simulink model "decentralized"  (R2017a)
settings: Solver=VariableStepAuto  StartTime=0.0  StopTime=6.01  RelTol=1e-3
values from neighbouring files (symbols this model uses):
  Kd = diag (Kd)    [calcula_ganhos.m]    (also in trajectoria_final.mat = [10.6713619257 0 0 0 0 0 0 10.022937202 0 0 0 0 ... (36 elem; trajectoria_final_2speed.mat = [10.6713619257 0 0 0 0 0 0 10.022937202 0 0 0 0 ... (36 elem; trajectoria_final_maxspeed.mat = [10.6713619257 0 0 0 0 0 0 10.022937202 0 0 0 0 ... (36 elem)
  Kp = diag (Kp)    [calcula_ganhos.m]    (also in trajectoria_final.mat = [67.0501444592 0 0 0 0 0 0 62.9759717625 0 0 0 0 ... (36 ele; trajectoria_final_2speed.mat = [67.0501444592 0 0 0 0 0 0 62.9759717625 0 0 0 0 ... (36 ele; trajectoria_final_maxspeed.mat = [67.0501444592 0 0 0 0 0 0 62.9759717625 0 0 0 0 ... (36 ele)
  q0 = [1.382 1.2 0.2 -0.5 0.4 0.34]'    [linear_trajectoryP.m]    (also in trajectoria_final.mat = [1.382 1.2 0.2 -0.5 0.4 0.34]; trajectoria_final_2speed.mat = [1.382 1.2 0.2 -0.5 0.4 0.34]; trajectoria_final_maxspeed.mat = [1.382 1.2 0.2 -0.5 0.4 0.34])
libraries: simulink x18, UR3_Lib x3, dspindex x2, sharedtransform x1, dspinverses x1
settings Model: Creator=dscat  LastModifiedBy=dscat

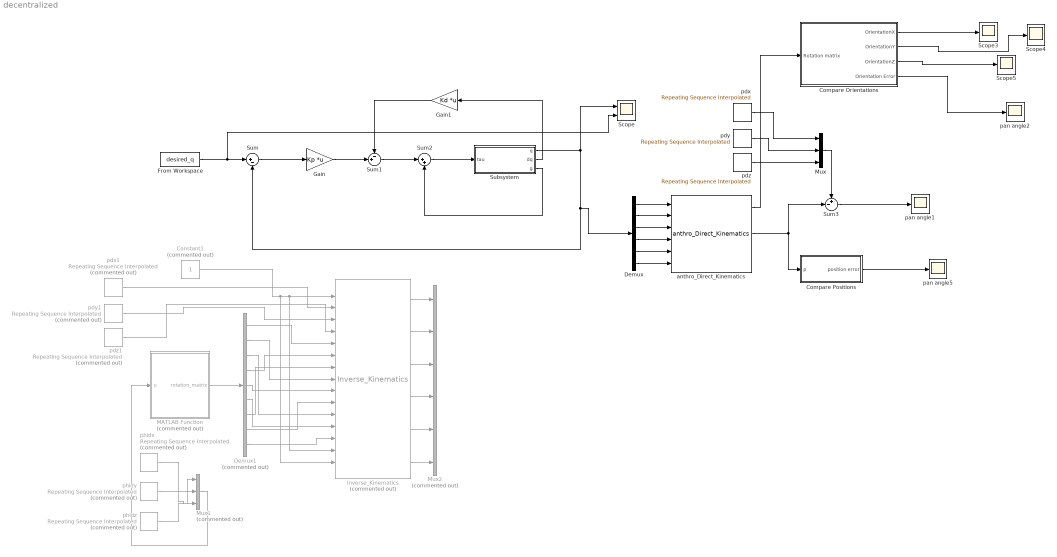
== system decentralized ==
  Compare Orientations : Subsystem
  Compare Positions : Subsystem
  Constant1 : Constant  Commented=on
  Demux : Demux  Outputs=6
  Demux1 : Demux  Commented=on  Outputs=9
  From Workspace : FromWorkspace  VariableName=desired_q  OutDataTypeStr=double  SampleTime=0
  Gain : Gain  Gain=Kp  Multiplication=Matrix(K*u)
  Gain1 : Gain  Gain=Kd  Multiplication=Matrix(K*u)
  Inverse_Kinematics : UR3_Lib/Inverse_Kinematics  Commented=on
  MATLAB Function : MATLAB Function  Commented=on  TreatAsAtomicUnit=on
  Mux : Mux  Inputs=3
  Mux1 : Mux  Commented=on  Inputs=3
  Mux2 : Mux  Commented=on  Inputs=6
  Scope : Scope  NumInputPorts=2
  Scope3 : Scope
  Scope4 : Scope
  Scope5 : Scope
  Subsystem : Subsystem
  Sum : Sum  Inputs=|+-
  Sum1 : Sum  Inputs=-+|
  Sum2 : Sum  Inputs=|++
  Sum3 : Sum  Inputs=+-|
  anthro_Direct_Kinematics : UR3_Lib/anthro_Direct_Kinematics
  pan angle1 : Scope
  pan angle2 : Scope
  pan angle5 : Scope
  pdx : simulink/Sources/Repeating Sequence Interpolated  OutValues=pdx  TimeValues=t  LookUpMeth=Interpolation-Use End Values  tsamp=0.01  OutMin=[]  OutMax=[]  OutDataTypeStr=double  OutputDataTypeScalingMode=double  OutDataType=fixdt(0,8)  OutScaling=2^-10
  pdx1 : simulink/Sources/Repeating Sequence Interpolated  Commented=on  OutValues=pdx  TimeValues=t  LookUpMeth=Interpolation-Use End Values  tsamp=0.01  OutMin=[]  OutMax=[]  OutDataTypeStr=double  OutputDataTypeScalingMode=double  OutDataType=fixdt(0,8)  OutScaling=2^-10
  pdy : simulink/Sources/Repeating Sequence Interpolated  OutValues=pdy  TimeValues=t  LookUpMeth=Interpolation-Use End Values  tsamp=0.01  OutMin=[]  OutMax=[]  OutDataTypeStr=double  OutputDataTypeScalingMode=double  OutDataType=fixdt(0,8)  OutScaling=2^-10
  pdy1 : simulink/Sources/Repeating Sequence Interpolated  Commented=on  OutValues=pdy  TimeValues=t  LookUpMeth=Interpolation-Use End Values  tsamp=0.01  OutMin=[]  OutMax=[]  OutDataTypeStr=double  OutputDataTypeScalingMode=double  OutDataType=fixdt(0,8)  OutScaling=2^-10
  pdz : simulink/Sources/Repeating Sequence Interpolated  OutValues=pdz  TimeValues=t  LookUpMeth=Interpolation-Use End Values  tsamp=0.01  OutMin=[]  OutMax=[]  OutDataTypeStr=double  OutputDataTypeScalingMode=double  OutDataType=fixdt(0,8)  OutScaling=2^-10
  pdz1 : simulink/Sources/Repeating Sequence Interpolated  Commented=on  OutValues=pdz  TimeValues=t  LookUpMeth=Interpolation-Use End Values  tsamp=0.01  OutMin=[]  OutMax=[]  OutDataTypeStr=double  OutputDataTypeScalingMode=double  OutDataType=fixdt(0,8)  OutScaling=2^-10
  phidx : simulink/Sources/Repeating Sequence Interpolated  Commented=on  OutValues=phidx  TimeValues=t  LookUpMeth=Interpolation-Use End Values  tsamp=0.01  OutMin=[]  OutMax=[]  OutDataTypeStr=double  OutputDataTypeScalingMode=double  OutDataType=fixdt(0,8)  OutScaling=2^-10
  phidy : simulink/Sources/Repeating Sequence Interpolated  Commented=on  OutValues=phidy  TimeValues=t  LookUpMeth=Interpolation-Use End Values  tsamp=0.01  OutMin=[]  OutMax=[]  OutDataTypeStr=double  OutputDataTypeScalingMode=double  OutDataType=fixdt(0,8)  OutScaling=2^-10
  phidz : simulink/Sources/Repeating Sequence Interpolated  Commented=on  OutValues=phidz  TimeValues=t  LookUpMeth=Interpolation-Use End Values  tsamp=0.01  OutMin=[]  OutMax=[]  OutDataTypeStr=double  OutputDataTypeScalingMode=double  OutDataType=fixdt(0,8)  OutScaling=2^-10
  wires:
  Sum/1 -> Gain/1
  Gain/1 -> Sum1/2
  Sum1/1 -> Sum2/1
  Sum2/1 -> Subsystem/1(tau)
  Subsystem/3(g) -> Sum2/2
  Subsystem/2(dq) -> Gain1/1
  Gain1/1 -> Sum1/1
  Subsystem/1(q) -> Demux/1, Sum/2, Scope/1
  From Workspace/1 -> Sum/1, Scope/2
  pdy/1 -> Mux/2
  pdx/1 -> Mux/1
  pdz/1 -> Mux/3
  Demux/1 -> anthro_Direct_Kinematics/1
  Demux/2 -> anthro_Direct_Kinematics/2
  Demux/3 -> anthro_Direct_Kinematics/3
  Demux/4 -> anthro_Direct_Kinematics/4
  Demux/5 -> anthro_Direct_Kinematics/5
  Demux/6 -> anthro_Direct_Kinematics/6
  anthro_Direct_Kinematics/2 -> Compare Positions/1("p "), Sum3/2
  Mux/1 -> Sum3/1
  Sum3/1 -> pan angle1/1
  Compare Positions/1(position error) -> pan angle5/1
  anthro_Direct_Kinematics/1 -> Compare Orientations/1("Rotation matrix ")
  Compare Orientations/1(OrientationX) -> Scope3/1
  Compare Orientations/2(OrientationY) -> Scope4/1
  Compare Orientations/4(Orientation Error) -> pan angle2/1
  Compare Orientations/3(OrientationZ) -> Scope5/1
  MATLAB Function/1(rotation_matrix) -> Demux1/1
  Demux1/1 -> Inverse_Kinematics/5
  Demux1/2 -> Inverse_Kinematics/8
  Demux1/3 -> Inverse_Kinematics/11
  Demux1/4 -> Inverse_Kinematics/6
  Demux1/5 -> Inverse_Kinematics/9
  Demux1/6 -> Inverse_Kinematics/12
  Demux1/7 -> Inverse_Kinematics/7
  Demux1/8 -> Inverse_Kinematics/10
  Demux1/9 -> Inverse_Kinematics/13
  Constant1/1 -> Inverse_Kinematics/15, Inverse_Kinematics/14, Inverse_Kinematics/1
  pdx1/1 -> Inverse_Kinematics/2
  pdz1/1 -> Inverse_Kinematics/4
  pdy1/1 -> Inverse_Kinematics/3
  phidx/1 -> Mux1/3
  phidy/1 -> Mux1/2
  phidz/1 -> Mux1/1
  Mux1/1 -> MATLAB Function/1(u)
  Inverse_Kinematics/6 -> Mux2/6
  Inverse_Kinematics/5 -> Mux2/5
  Inverse_Kinematics/4 -> Mux2/4
  Inverse_Kinematics/2 -> Mux2/2
  Inverse_Kinematics/3 -> Mux2/3
  Inverse_Kinematics/1 -> Mux2/1

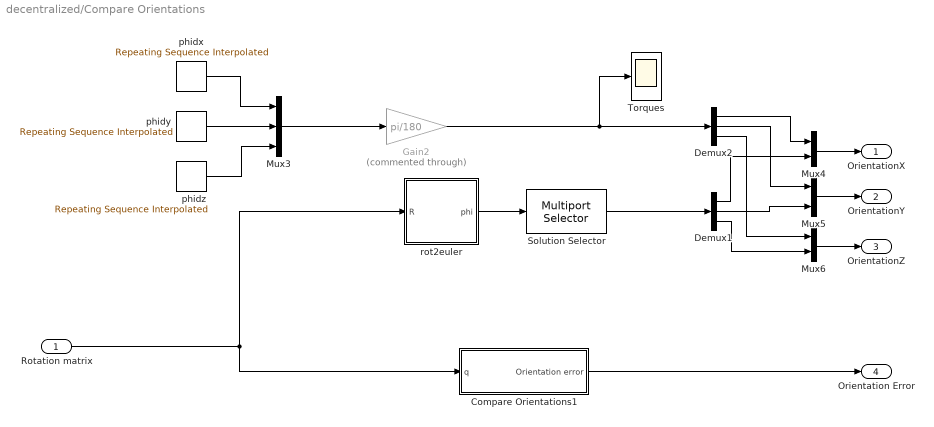
== system decentralized/Compare Orientations ==
  "Rotation matrix " : Inport
  Compare Orientations1 : Subsystem
  Demux1 : Demux  Outputs=3
  Demux2 : Demux  Outputs=3
  Gain2 : Gain  Commented=through  Gain=pi/180
  Mux3 : Mux  Inputs=3
  Mux4 : Mux  Inputs=2
  Mux5 : Mux  Inputs=2
  Mux6 : Mux  Inputs=2
  Solution Selector : dspindex/Multiport Selector  rowsOrCols=Columns  idxCellArray=1  idxErrMode=Clip Index
  Torques : Scope
  phidx : simulink/Sources/Repeating Sequence Interpolated  OutValues=phidx  TimeValues=t  LookUpMeth=Interpolation-Use End Values  tsamp=0.01  OutMin=[]  OutMax=[]  OutDataTypeStr=double  OutputDataTypeScalingMode=double  OutDataType=fixdt(0,8)  OutScaling=2^-10
  phidy : simulink/Sources/Repeating Sequence Interpolated  OutValues=phidy  TimeValues=t  LookUpMeth=Interpolation-Use End Values  tsamp=0.01  OutMin=[]  OutMax=[]  OutDataTypeStr=double  OutputDataTypeScalingMode=double  OutDataType=fixdt(0,8)  OutScaling=2^-10
  phidz : simulink/Sources/Repeating Sequence Interpolated  OutValues=phidz  TimeValues=t  LookUpMeth=Interpolation-Use End Values  tsamp=0.01  OutMin=[]  OutMax=[]  OutDataTypeStr=double  OutputDataTypeScalingMode=double  OutDataType=fixdt(0,8)  OutScaling=2^-10
  rot2euler : MATLAB Function  TreatAsAtomicUnit=on
  OrientationX : Outport
  OrientationY : Outport  Port=2
  OrientationZ : Outport  Port=3
  Orientation Error : Outport  Port=4
  wires:
  Gain2/1 -> Demux2/1, Torques/1
  Compare Orientations1/1(Orientation error) -> Orientation Error/1
  phidx/1 -> Mux3/1
  Mux3/1 -> Gain2/1
  phidz/1 -> Mux3/3
  phidy/1 -> Mux3/2
  Mux6/1 -> OrientationZ/1
  Mux5/1 -> OrientationY/1
  Mux4/1 -> OrientationX/1
  Demux2/3 -> Mux6/1
  Demux2/2 -> Mux5/1
  Demux2/1 -> Mux4/1
  Demux1/1 -> Mux4/2
  Solution Selector/1 -> Demux1/1
  rot2euler/1(phi) -> Solution Selector/1
  Demux1/3 -> Mux6/2
  Demux1/2 -> Mux5/2
  "Rotation matrix "/1 -> Compare Orientations1/1("q "), rot2euler/1(R)

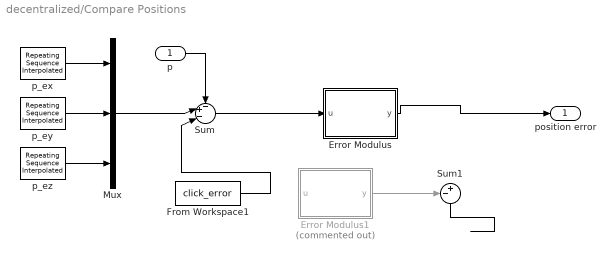
== system decentralized/Compare Positions ==
  "p " : Inport
  Error Modulus : MATLAB Function  TreatAsAtomicUnit=on
  Error Modulus1 : MATLAB Function  Commented=on  TreatAsAtomicUnit=on
  From Workspace1 : FromWorkspace  VariableName=click_error  OutDataTypeStr=double  SampleTime=0
  Mux : Mux  Inputs=3
  Sum : Sum  Inputs=-+-|
  Sum1 : Sum  Inputs=-+|
  p_ex : simulink/Sources/Repeating Sequence Interpolated  OutValues=pdx  TimeValues=t  LookUpMeth=Interpolation-Use End Values  tsamp=0.01  OutMin=[]  OutMax=[]  OutDataTypeStr=double  OutputDataTypeScalingMode=double  OutDataType=fixdt(0,8)  OutScaling=2^-10
  p_ey : simulink/Sources/Repeating Sequence Interpolated  OutValues=pdy  TimeValues=t  LookUpMeth=Interpolation-Use End Values  tsamp=0.01  OutMin=[]  OutMax=[]  OutDataTypeStr=double  OutputDataTypeScalingMode=double  OutDataType=fixdt(0,8)  OutScaling=2^-10
  p_ez : simulink/Sources/Repeating Sequence Interpolated  OutValues=pdz  TimeValues=t  LookUpMeth=Interpolation-Use End Values  tsamp=0.01  OutMin=[]  OutMax=[]  OutDataTypeStr=double  OutputDataTypeScalingMode=double  OutDataType=fixdt(0,8)  OutScaling=2^-10
  position error : Outport
  wires:
  Sum/1 -> Error Modulus/1(u)
  "p "/1 -> Sum/1
  Error Modulus/1(y) -> position error/1
  Mux/1 -> Sum/2
  p_ez/1 -> Mux/3
  p_ey/1 -> Mux/2
  p_ex/1 -> Mux/1
  From Workspace1/1 -> Sum/3
  Error Modulus1/1(y) -> Sum1/1
  Sum1/1 -> ?

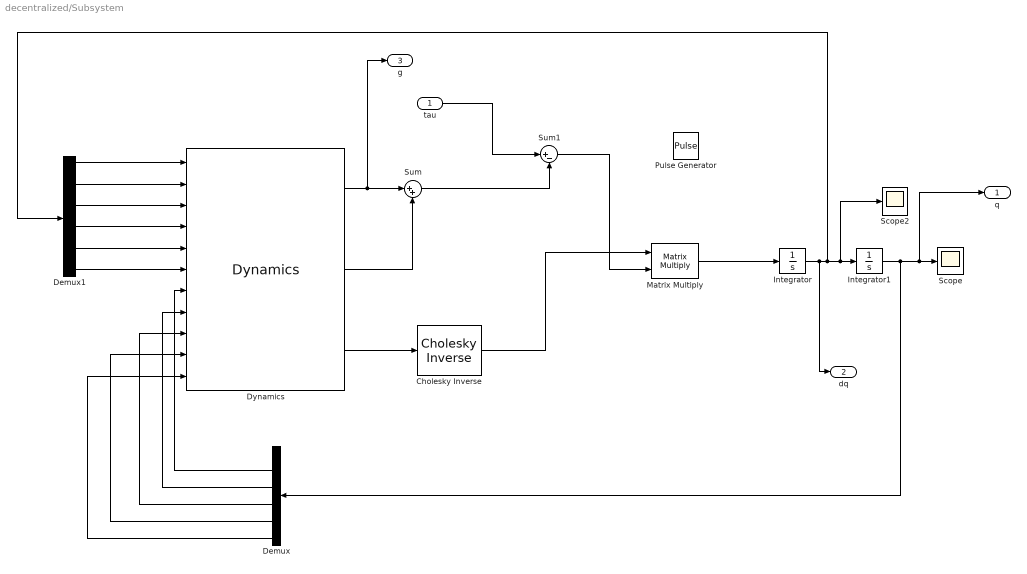
== system decentralized/Subsystem ==
  tau : Inport
  Cholesky Inverse : dspinverses/Cholesky Inverse  errmode=Warning
      settings: SourceProductName=DSP System Toolbox  SourceProductBaseCode=DS
  Demux : Demux  Outputs=6
  Demux1 : Demux  Outputs=6
  Dynamics : UR3_Lib/Dynamics
  Integrator : Integrator  InitialCondition=[0 0 0 0 0 0]'
  Integrator1 : Integrator  InitialCondition=q0
  Matrix Multiply : Product  Multiplication=Matrix(*)
  Pulse Generator : DiscretePulseGenerator  PulseType=Time based  Amplitude=[1 0 0 0 0 0]  Period=3  PulseWidth=5
  Scope : Scope
  Scope2 : Scope
  Sum : Sum  Inputs=|++
  Sum1 : Sum  Inputs=|+-
  q : Outport
  dq : Outport  Port=2
  g : Outport  Port=3
  wires:
  tau/1 -> Sum1/1
  Demux/3 -> Dynamics/8
  Demux/5 -> Dynamics/10
  Demux1/3 -> Dynamics/3
  Demux1/4 -> Dynamics/4
  Demux1/2 -> Dynamics/2
  Demux1/5 -> Dynamics/5
  Demux/2 -> Dynamics/7
  Demux/4 -> Dynamics/9
  Demux1/6 -> Dynamics/6
  Matrix Multiply/1 -> Integrator/1
  Sum1/1 -> Matrix Multiply/2
  Dynamics/3 -> Cholesky Inverse/1
  Demux/6 -> Dynamics/11
  Dynamics/1 -> g/1, Sum/1
  Cholesky Inverse/1 -> Matrix Multiply/1
  Integrator/1 -> dq/1, Demux1/1, Scope2/1, Integrator1/1
  Sum/1 -> Sum1/2
  Dynamics/2 -> Sum/2
  Demux1/1 -> Dynamics/1
  Integrator1/1 -> Demux/1, q/1, Scope/1

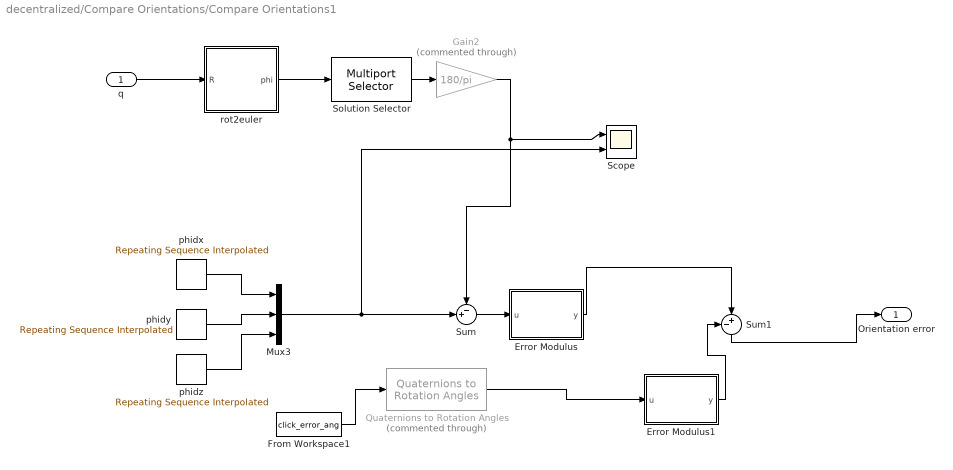
== system decentralized/Compare Orientations/Compare Orientations1 ==
  "q " : Inport
  Error Modulus : MATLAB Function  TreatAsAtomicUnit=on
  Error Modulus1 : MATLAB Function  TreatAsAtomicUnit=on
  From Workspace1 : FromWorkspace  VariableName=click_error_ang  OutDataTypeStr=double  SampleTime=0
  Gain2 : Gain  Commented=through  Gain=180/pi
  Mux3 : Mux  Inputs=3
  Quaternions to Rotation Angles : sharedtransform/Quaternions to Rotation Angles  Commented=through  rotationOrder=ZYX
  Scope : Scope  NumInputPorts=2
  Solution Selector : dspindex/Multiport Selector  rowsOrCols=Columns  idxCellArray=1  idxErrMode=Clip Index
  Sum : Sum  Inputs=-+|
  Sum1 : Sum  Inputs=-+|
  phidx : simulink/Sources/Repeating Sequence Interpolated  OutValues=phidx  TimeValues=t  LookUpMeth=Interpolation-Use End Values  tsamp=0.01  OutMin=[]  OutMax=[]  OutDataTypeStr=double  OutputDataTypeScalingMode=double  OutDataType=fixdt(0,8)  OutScaling=2^-10
  phidy : simulink/Sources/Repeating Sequence Interpolated  OutValues=phidy  TimeValues=t  LookUpMeth=Interpolation-Use End Values  tsamp=0.01  OutMin=[]  OutMax=[]  OutDataTypeStr=double  OutputDataTypeScalingMode=double  OutDataType=fixdt(0,8)  OutScaling=2^-10
  phidz : simulink/Sources/Repeating Sequence Interpolated  OutValues=phidz  TimeValues=t  LookUpMeth=Interpolation-Use End Values  tsamp=0.01  OutMin=[]  OutMax=[]  OutDataTypeStr=double  OutputDataTypeScalingMode=double  OutDataType=fixdt(0,8)  OutScaling=2^-10
  rot2euler : MATLAB Function  TreatAsAtomicUnit=on
  Orientation error : Outport
  wires:
  Error Modulus/1(y) -> Sum1/2
  Gain2/1 -> Scope/1, Sum/1
  Sum/1 -> Error Modulus/1(u)
  Mux3/1 -> Sum/2, Scope/2
  Solution Selector/1 -> Gain2/1
  phidx/1 -> Mux3/1
  "q "/1 -> rot2euler/1(R)
  phidz/1 -> Mux3/3
  phidy/1 -> Mux3/2
  rot2euler/1(phi) -> Solution Selector/1
  From Workspace1/1 -> Quaternions to Rotation Angles/1
  Quaternions to Rotation Angles/1 -> Error Modulus1/1(u)
  Error Modulus1/1(y) -> Sum1/1
  Sum1/1 -> Orientation error/1

== matlab function decentralized/Compare Orientations/Compare Orientations1/Error Modulus ==
  data: u input; y output
function y = Norm(u)
%#codegen

y = norm (u);

== matlab function decentralized/Compare Orientations/Compare Orientations1/Error Modulus1 ==
  data: u input; y output
function y = Norm(u)
%#codegen

y = norm (u);

== matlab function decentralized/MATLAB Function ==
  data: u input; rotation_matrix output
function rotation_matrix = euler_rotationm(u)

rotation_matrix = eul2rotm(u);

== matlab function decentralized/Compare Orientations/Compare Orientations1/rot2euler ==
  data: R input; phi output
function phi   = Rot2Euler( R )
%This function converts the rotation matrix into Quarternion Representation
phi=zeros(3,2);

%phi_y6 € ]-pi/2,pi/2[
phi(1,1)=atan2(R(2,1),R(1,1));
phi(2,1)=atan2(-R(3,1),sqrt(R(3,2)^2+R(3,3)^2));
phi(3,1)=atan2(R(3,2),R(3,3));
%q6 € ]pi/2,3pi/2[
phi(1,2)=atan2(-R(2,1),-R(1,1));
phi(2,2)=atan2(-R(3,1),-sqrt(R(3,2)^2+R(3,3)^2));
phi(3,2)=atan2(-R(3,2),-R(3,3));

end

== matlab function decentralized/Compare Positions/Error Modulus1 ==
  data: u input; y output
function y = Norm(u)
%#codegen

y = norm (u);

== matlab function decentralized/Compare Orientations/rot2euler ==
  data: R input; phi output
function phi   = Rot2Euler( R )
%This function converts the rotation matrix into Quarternion Representation
phi=zeros(3,2);

%phi_y6 € ]-pi/2,pi/2[
phi(1,1)=atan2(R(2,1),R(1,1));
phi(2,1)=atan2(-R(3,1),sqrt(R(3,2)^2+R(3,3)^2));
phi(3,1)=atan2(R(3,2),R(3,3));
%q6 € ]pi/2,3pi/2[
phi(1,2)=atan2(-R(2,1),-R(1,1));
phi(2,2)=atan2(-R(3,1),-sqrt(R(3,2)^2+R(3,3)^2));
phi(3,2)=atan2(-R(3,2),-R(3,3));

end

== matlab function decentralized/Compare Positions/Error Modulus ==
  data: u input; y output
function y = Norm(u)
%#codegen

y = norm (u);
